simulink model "scheme1"  (R2014a)
settings: Solver=ode45  StartTime=0.0  StopTime=10  MaxStep=0.001  MinStep=0.0001  RelTol=1e-3
settings Model: Creator=Valentin  LastModifiedBy=Анастасия

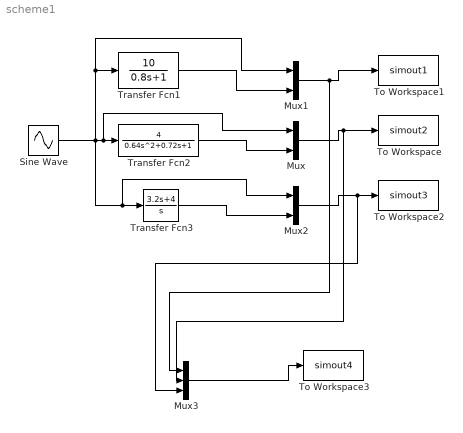
== system scheme1 ==
  Mux : Mux  Inputs=2
  Mux1 : Mux  Inputs=2
  Mux2 : Mux  Inputs=2
  Mux3 : Mux  Inputs=3
  Sine Wave : Sin  Frequency=100  SampleTime=0
  To Workspace : ToWorkspace  VariableName=simout2  SaveFormat=Timeseries  SampleTime=-1
  To Workspace1 : ToWorkspace  VariableName=simout1  SaveFormat=Timeseries  SampleTime=-1
  To Workspace2 : ToWorkspace  VariableName=simout3  SaveFormat=Timeseries  SampleTime=-1
  To Workspace3 : ToWorkspace  VariableName=simout4  SaveFormat=Timeseries  SampleTime=-1
  Transfer Fcn1 : TransferFcn  Numerator=[10]  Denominator=[0.8 1]
  Transfer Fcn2 : TransferFcn  Numerator=[4]  Denominator=[0.64 0.72 1]
  Transfer Fcn3 : TransferFcn  Numerator=[3.2 4]  Denominator=[1 0]
  wires:
  Mux/1 -> Mux3/2, To Workspace/1
  Transfer Fcn2/1 -> Mux/2
  Mux1/1 -> Mux3/1, To Workspace1/1
  Transfer Fcn1/1 -> Mux1/2
  Sine Wave/1 -> Mux2/1, Transfer Fcn3/1, Mux1/1, Transfer Fcn1/1, Mux/1, Transfer Fcn2/1
  Mux2/1 -> Mux3/3, To Workspace2/1
  Transfer Fcn3/1 -> Mux2/2
  Mux3/1 -> To Workspace3/1
